simulink library "algebraicManip_lib"  (R2025a)
settings: Solver=VariableStepAuto  StartTime=0.0  StopTime=10.0  RelTol=1e-3
settings Model: Creator=mbhattu  LastModifiedBy=mbhattu

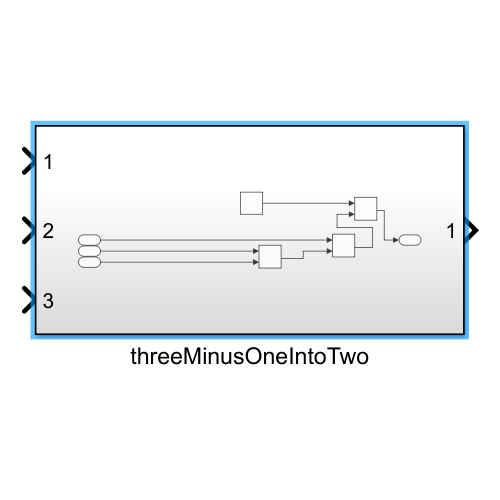
[thumbnail: Simulink's stored preview of the top-level diagram]
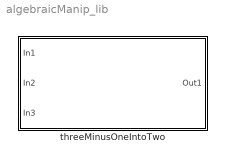
== system algebraicManip_lib ==
  threeMinusOneIntoTwo : Subsystem

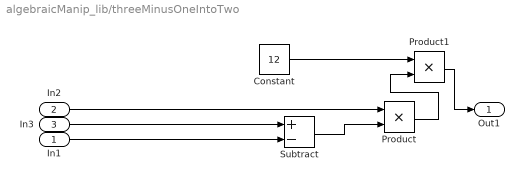
== system algebraicManip_lib/threeMinusOneIntoTwo ==
  In1 : Inport
  In2 : Inport  Port=2
  In3 : Inport  Port=3
  Constant : Constant  Value=12
  Product : Product
  Product1 : Product
  Subtract : Sum  Inputs=+-
  Out1 : Outport
  wires:
  In1/1 -> Subtract/2
  In3/1 -> Subtract/1
  In2/1 -> Product/1
  Subtract/1 -> Product/2
  Product/1 -> Product1/2
  Constant/1 -> Product1/1
  Product1/1 -> Out1/1
